simulink model "UAV_Task4_3"  (R2024b)
settings: Solver=ode45  StartTime=0  StopTime=100  RelTol=1e-5  AbsTol=1e-5
values from neighbouring files (symbols this model uses):
  adaptiveActivation = 1    [UAV_Task4_1_main.m]    (also in UAV_Task4_2_main.m = 0; UAV_Task4_3_main.m)
  B_p = 1/UAV.m    [UAV_Task4_1_main.m]    (also in UAV_Task4_2_main.m; UAV_Task4_3_main.m)
  F2plus = F2'*pinv(F2*F2')    [UAV_Task4_1_main.m]    (also in UAV_Task4_2_main.m; UAV_Task4_3_main.m)
  fe_0 = [0;0]    [UAV_Task4_3_main.m]
  Gamma_a = 1*[1 1 1 1]'    [UAV_Task4_1_main.m]    (also in UAV_Task4_2_main.m; UAV_Task4_3_main.m = 1*[1 1 1 1 1 1]')
  Gamma_a_scalar = 1    [UAV_Task4_2_main.m]    (also in UAV_Task4_3_main.m)
  gravityInAdaptiveController = 1    [UAV_Task4_1_main.m]    (also in UAV_Task4_2_main.m; UAV_Task4_3_main.m)
  k_f = 0.3379e-6    (= 3.379e-07)    [UAV_Task4_1_main.m]    (also in UAV_Task4_2_main.m; UAV_Task4_3_main.m)
  L = 10    [UAV_Task4_1_main.m]    (also in UAV_Task4_2_main.m; UAV_Task4_3_main.m)
  lambda_0 = 1    [UAV_Task4_1_main.m]    (also in UAV_Task4_2_main.m; UAV_Task4_3_main.m)
  Omega_0 = [1500 1500 1500 1500]'    [UAV_Task4_1_main.m]    (also in UAV_Task4_2_main.m; UAV_Task4_3_main.m)
  omegab_0 = [0; 0; 0]    [UAV_Task4_1_main.m]    (also in UAV_Task4_2_main.m; UAV_Task4_3_main.m)
  p_0 = [0; 0; 0]    [UAV_Task4_1_main.m]    (also in UAV_Task4_2_main.m; UAV_Task4_3_main.m)
  PO = 1    [UAV_Task4_1_main.m]    (also in UAV_Task4_2_main.m; UAV_Task4_3_main.m)
  q_0 = eul2quat([0, 0, 0]*degToRad,'ZYX')'    [UAV_Task4_1_main.m]    (also in UAV_Task4_2_main.m; UAV_Task4_3_main.m)
  scenario = 2    [UAV_Task4_1_main.m]    (also in UAV_Task4_2_main.m; UAV_Task4_3_main.m)
  theta_0 = [0.07;0.07;0.1]    [UAV_Task4_1_main.m]    (also in UAV_Task4_2_main.m; UAV_Task4_3_main.m)
  vb_0 = [0; 0; 0]    [UAV_Task4_1_main.m]    (also in UAV_Task4_2_main.m; UAV_Task4_3_main.m)
undefined symbols (not defined in the file or in its folder): adaptive_controller, ctrl, D_fv_i, dyn, e_3, epsilon_PO, fw_params_fc, g, lambda_i, par, pos, pos_pp, projection_operator, targetParams, theta_M, UAV, v_M, vel, vel_pp
libraries: slpidlib x22, matrix_library x6, aerolibutil x2, uavutilslib x1
(part 4 of 4)

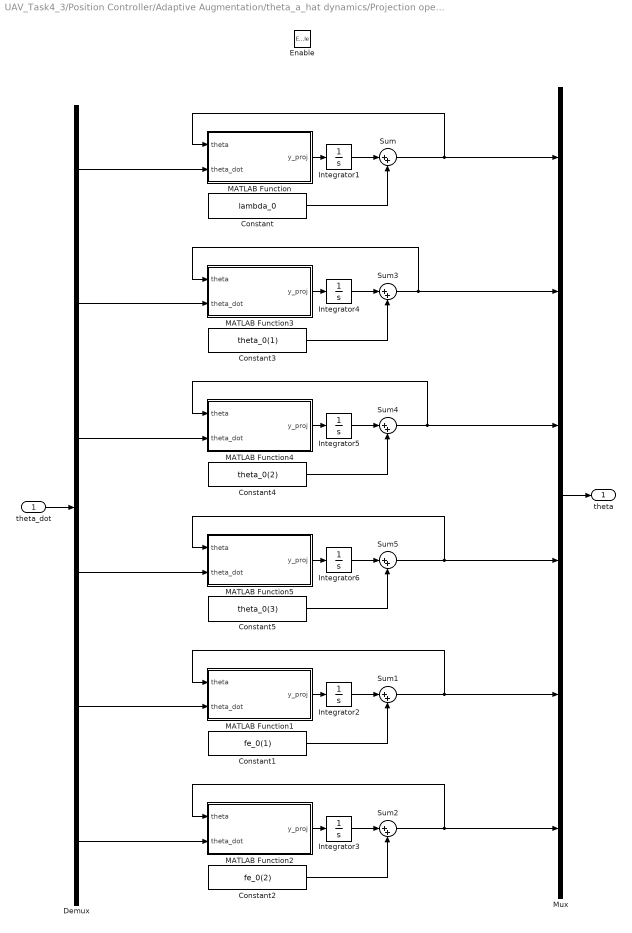
== system UAV_Task4_3/Position Controller/Adaptive Augmentation/theta_a_hat dynamics/Projection operator ==
  theta_dot : Inport
  Enable : EnablePort
  Constant : Constant  Value=lambda_0
  Constant1 : Constant  Value=fe_0(1)
  Constant2 : Constant  Value=fe_0(2)
  Constant3 : Constant  Value=theta_0(1)
  Constant4 : Constant  Value=theta_0(2)
  Constant5 : Constant  Value=theta_0(3)
  Demux : Demux  Outputs=6
  Integrator{1..6} (6 alike) : Integrator
  MATLAB Function : MATLAB Function  TreatAsAtomicUnit=on
  MATLAB Function1 : MATLAB Function  TreatAsAtomicUnit=on
  MATLAB Function2 : MATLAB Function  TreatAsAtomicUnit=on
  MATLAB Function3 : MATLAB Function  TreatAsAtomicUnit=on
  MATLAB Function4 : MATLAB Function  TreatAsAtomicUnit=on
  MATLAB Function5 : MATLAB Function  TreatAsAtomicUnit=on
  Mux : Mux  Inputs=6
  Sum{,1..5} (6 alike) : Sum  Inputs=|++
  theta : Outport
  wires:
  MATLAB Function/1(y_proj) -> Integrator1/1
  Sum/1 -> MATLAB Function/1(theta), Mux/1
  Integrator1/1 -> Sum/1
  Constant/1 -> Sum/2
  Demux/1 -> MATLAB Function/2(theta_dot)
  theta_dot/1 -> Demux/1
  Constant3/1 -> Sum3/2
  MATLAB Function3/1(y_proj) -> Integrator4/1
  Sum3/1 -> MATLAB Function3/1(theta), Mux/2
  Integrator4/1 -> Sum3/1
  Demux/2 -> MATLAB Function3/2(theta_dot)
  Constant4/1 -> Sum4/2
  MATLAB Function4/1(y_proj) -> Integrator5/1
  Sum4/1 -> MATLAB Function4/1(theta), Mux/3
  Integrator5/1 -> Sum4/1
  Demux/3 -> MATLAB Function4/2(theta_dot)
  Constant5/1 -> Sum5/2
  MATLAB Function5/1(y_proj) -> Integrator6/1
  Sum5/1 -> MATLAB Function5/1(theta), Mux/4
  Integrator6/1 -> Sum5/1
  Demux/4 -> MATLAB Function5/2(theta_dot)
  Mux/1 -> theta/1
  MATLAB Function1/1(y_proj) -> Integrator2/1
  Sum1/1 -> MATLAB Function1/1(theta), Mux/5
  Integrator2/1 -> Sum1/1
  Demux/5 -> MATLAB Function1/2(theta_dot)
  Constant1/1 -> Sum1/2
  MATLAB Function2/1(y_proj) -> Integrator3/1
  Sum2/1 -> Mux/6, MATLAB Function2/1(theta)
  Integrator3/1 -> Sum2/1
  Demux/6 -> MATLAB Function2/2(theta_dot)
  Constant2/1 -> Sum2/2

== system UAV_Task4_3/POSITION + ADAPTIVE CONTROLLER/Subsystem1/Subsystem1/Adaptive Augmentation/Predictor (x_p_hat) dynamics ==
  Lambda_hat : Inport
  u : Inport  Port=2
  phi_p : Inport  Port=3
  theta_p_hat : Inport  Port=4
  x_p : Inport  Port=5
  Add : Sum
  Constant : Constant  Value=g*e3
  Gain : Gain  Gain=B_p  Multiplication=Matrix(K*u)
  Gain1 : Gain  Gain=L
  Gain2 : Gain  Gain=gravityInAdaptiveController
  Gain3 : Gain
  Integrator : Integrator  InitialCondition=vb_0
  Matrix Multiply : Product
  Matrix Multiply1 : Product  Multiplication=Matrix(*)
  Reshape : Reshape  OutputDimensionality=Column vector (2-D)
  Reshape1 : Reshape  OutputDimensionality=Column vector (2-D)
  Reshape2 : Reshape  OutputDimensionality=Column vector (2-D)
  Scope : Scope
  Scope1 : Scope
  Sum : Sum  Inputs=+++
  Sum1 : Sum  Inputs=-+|
  Transpose : Math  Operator=transpose
  x_p_hat : Outport
  wires:
  Lambda_hat/1 -> Matrix Multiply/1
  Matrix Multiply/1 -> Add/1
  phi_p/1 -> Transpose/1
  theta_p_hat/1 -> Matrix Multiply1/2
  Matrix Multiply1/1 -> Add/2
  Add/1 -> Gain/1
  Gain/1 -> Reshape1/1
  Gain1/1 -> Reshape/1
  x_p/1 -> Scope1/1, Sum1/2
  Sum1/1 -> Gain1/1
  Integrator/1 -> Scope/1, Sum1/1, x_p_hat/1
  Sum/1 -> Integrator/1
  Reshape/1 -> Sum/1
  Reshape1/1 -> Sum/2
  Reshape2/1 -> Sum/3
  Constant/1 -> Gain2/1
  Transpose/1 -> Matrix Multiply1/1
  u/1 -> Matrix Multiply/2
  Gain2/1 -> Gain3/1
  Gain3/1 -> Reshape2/1

== system UAV_Task4_3/POSITION + ADAPTIVE CONTROLLER/Subsystem1/Subsystem1/Adaptive Augmentation/Subsystem ==
  Lambda_hat : Inport
  u_b : Inport  Port=2
  phi_p : Inport  Port=3
  theta_p_hat : Inport  Port=4
  Constant : Constant  Value=eye(3,3)
  Gain : Gain  Commented=through  Gain=-1
  Gain1 : Gain
  Inverse : MATLAB Function  TreatAsAtomicUnit=on
  Product : Product  Multiplication=Matrix(*)
  Product1 : Product  Inputs=3  Multiplication=Matrix(*)
  Subtract : Sum  Inputs=-+
  Subtract1 : Sum  Inputs=+-
  Transpose : Math  Operator=transpose
  u_a : Outport
  wires:
  Lambda_hat/1 -> Inverse/1(u)
  Inverse/1(y) -> Product1/1, Subtract/2
  Constant/1 -> Subtract/1
  Subtract/1 -> Product/1
  u_b/1 -> Product/2
  Product/1 -> Gain1/1
  Subtract1/1 -> u_a/1
  phi_p/1 -> Transpose/1
  Transpose/1 -> Gain/1
  theta_p_hat/1 -> Product1/3
  Product1/1 -> Subtract1/2
  Gain/1 -> Product1/2
  Gain1/1 -> Subtract1/1

== system UAV_Task4_3/POSITION + ADAPTIVE CONTROLLER/Subsystem1/Subsystem1/Adaptive Augmentation/phi_a ==
  u : Inport
  phi_p : Inport  Port=2
  Matrix Concatenate : Concatenate  Mode=Multidimensional array
  Scope : Scope
  Transpose : Math  Operator=transpose
  phi_a : Outport
  wires:
  Matrix Concatenate/1 -> Scope/1, phi_a/1
  u/1 -> Transpose/1
  phi_p/1 -> Matrix Concatenate/2
  Transpose/1 -> Matrix Concatenate/1

== system UAV_Task4_3/POSITION + ADAPTIVE CONTROLLER/Subsystem1/Subsystem1/Adaptive Augmentation/phi_p ==
  x_p : Inport
  Create Diagonal Matrix : matrix_library/Create Diagonal Matrix
  Gain : Gain  Gain=-1
  phi_p : Outport
  wires:
  x_p/1 -> Gain/1
  Gain/1 -> Create Diagonal Matrix/1
  Create Diagonal Matrix/1 -> phi_p/1

== system UAV_Task4_3/POSITION + ADAPTIVE CONTROLLER/Subsystem1/Subsystem1/Adaptive Augmentation/theta_a_hat dynamics ==
  Gamma_a : Inport
  phi_a : Inport  Port=2
  B_p : Inport  Port=3
  x_p : Inport  Port=4
  x_p_hat : Inport  Port=5
  Constant1 : Constant  Value=PO
  Dot Product : DotProduct  OutDataTypeStr=Inherit: Inherit via internal rule
  Integrator : Integrator  InitialCondition=[lambda_0; theta_0]
  Matrix Multiply1 : Product
  Matrix Multiply2 : Product  Multiplication=Matrix(*)
  Matrix Multiply3 : Product
  Projection operator : Subsystem
  Scope{,1..4} (5 alike) : Scope
  Sqrt : Sqrt
  Subtract : Sum  Inputs=+-
  Switch : Switch  Criteria=u2 > Threshold  SaturateOnIntegerOverflow=off  InputSameDT=off
  To Workspace : ToWorkspace  VariableName=e_p_hat  SaveFormat=Timeseries  SampleTime=-1
  Transpose : Math  Operator=transpose
  Transpose1 : Math  Commented=through  Operator=transpose
  theta_a_hat : Outport
  wires:
  x_p_hat/1 -> Subtract/2
  B_p/1 -> Transpose/1
  Subtract/1 -> Scope4/1, Dot Product/2, Dot Product/1, Matrix Multiply1/2
  Transpose/1 -> Matrix Multiply1/1
  phi_a/1 -> Transpose1/1
  Matrix Multiply1/1 -> Scope3/1, Matrix Multiply2/2
  Gamma_a/1 -> Matrix Multiply3/1
  Matrix Multiply2/1 -> Matrix Multiply3/2
  Matrix Multiply3/1 -> Projection operator/1(theta_dot), Scope2/1, Integrator/1
  x_p/1 -> Subtract/1
  Constant1/1 -> Switch/2, Projection operator/Enable
  Integrator/1 -> Scope1/1, Switch/3
  Switch/1 -> theta_a_hat/1
  Projection operator/1(theta) -> Scope/1, Switch/1
  Dot Product/1 -> Sqrt/1
  Sqrt/1 -> To Workspace/1
  Transpose1/1 -> Matrix Multiply2/1

== system UAV_Task4_3/POSITION + ADAPTIVE CONTROLLER/Subsystem1/Subsystem1/Adaptive Augmentation/theta_a_hat dynamics/Projection operator ==
  theta_dot : Inport
  Enable : EnablePort
  Constant : Constant  Value=lambda_0
  Constant3 : Constant  Value=theta_0(1)
  Constant4 : Constant  Value=theta_0(2)
  Constant5 : Constant  Value=theta_0(3)
  Demux : Demux
  Integrator{1,4..6} (4 alike) : Integrator
  MATLAB Function : MATLAB Function  TreatAsAtomicUnit=on
  MATLAB Function3 : MATLAB Function  TreatAsAtomicUnit=on
  MATLAB Function4 : MATLAB Function  TreatAsAtomicUnit=on
  MATLAB Function5 : MATLAB Function  TreatAsAtomicUnit=on
  Mux : Mux
  Sum{,3..5} (4 alike) : Sum  Inputs=|++
  theta : Outport
  wires:
  MATLAB Function/1(y_proj) -> Integrator1/1
  Sum/1 -> MATLAB Function/1(theta), Mux/1
  Integrator1/1 -> Sum/1
  Constant/1 -> Sum/2
  Demux/1 -> MATLAB Function/2(theta_dot)
  theta_dot/1 -> Demux/1
  Constant3/1 -> Sum3/2
  MATLAB Function3/1(y_proj) -> Integrator4/1
  Sum3/1 -> Mux/2, MATLAB Function3/1(theta)
  Integrator4/1 -> Sum3/1
  Demux/2 -> MATLAB Function3/2(theta_dot)
  Constant4/1 -> Sum4/2
  MATLAB Function4/1(y_proj) -> Integrator5/1
  Sum4/1 -> Mux/3, MATLAB Function4/1(theta)
  Integrator5/1 -> Sum4/1
  Demux/3 -> MATLAB Function4/2(theta_dot)
  Constant5/1 -> Sum5/2
  MATLAB Function5/1(y_proj) -> Integrator6/1
  Sum5/1 -> MATLAB Function5/1(theta), Mux/4
  Integrator6/1 -> Sum5/1
  Demux/4 -> MATLAB Function5/2(theta_dot)
  Mux/1 -> theta/1

== matlab function UAV_Task4_3/POSITION + ADAPTIVE CONTROLLER/Subsystem1/Subsystem1/Adaptive Augmentation/Subsystem/Inverse ==
  data: u input; y output
function y = fcn(u)

Lambda = diag([u;u;u]);
y = inv(Lambda);

== matlab function UAV_Task4_3/Main Trajectory Generation ==
  data: v_b_dot output size=[3,1]; v_b output size=[3,1]; p output size=[3,1]; time input; omega_p_dot output size=[3,1]; omega_p output size=[3,1]; targetParams parameter; heading output; scenario parameter
function [v_b_dot, v_b, p, omega_p_dot, omega_p, heading]   = fcn(time, targetParams, scenario)

if scenario == 1
    omega_p_dot = targetParams.omega_p_dot;
    v_b_dot = targetParams.v_b_dot;
    omega_p = targetParams.omega_p;
    v_b = targetParams.v_b;
    p = targetParams.p;
    heading = targetParams.heading;
else
    radius = norm([sqrt(2)/2 5*sqrt(2)/2 -1]);
    angle = 2*pi/60*time;
    p = [radius*sin(angle); radius*cos(angle); -1];
    v_b = pi/30*radius*[cos(angle); -sin(angle); 0];
    v_b_dot = ((pi/30*radius)^2)/3*[-sin(angle); -cos(angle); 0];
    omega_p = [0; 0; 2*pi/60];
    omega_p_dot = [0; 0; 0];
    %heading = -angle;
    heading = 0;

    % f = pi/30;
    % p = [cos(f*time) sin(f*time) -1]';
    % v_b = [-f*sin(f*time) f*cos(f*time) 0]';
    % v_b_dot = [-f^2*cos(f*time) -f^2*sin(f*time) 0]';
end

== matlab function UAV_Task4_3/Plant Dynamics/Attitude kinematics&dynamics/MATLAB Function ==
  data: quat input; quat_M output
function quat_M = fcn(quat)
qs = quat(4);

quat_M = [qs;
          quat(1) ;
          quat(2) ;
          quat(3)];

== matlab function UAV_Task4_3/POSITION + ADAPTIVE CONTROLLER/Subsystem1/Subsystem1/Adaptive Augmentation/theta_a_hat dynamics/Projection operator/MATLAB Function ==
  data: theta input; y_proj output; theta_dot input; par parameter
function y_proj = proj(theta,theta_dot,par)

% I could get rid of the center by not feeding it to the function

Gamma = par.Gamma(1);
eps_proj = par.eps_proj;
theta_M = par.theta_M(1);
center = par.center(1);
theta = theta - center;

f = 1/(eps_proj*theta_M^2)*((1+eps_proj)*(theta')*theta-theta_M^2);
grad_f = 2/(eps_proj*theta_M^2)*(1+eps_proj)*theta;

if f>0 && all(theta_dot'*Gamma*grad_f>0)
    y_proj = Gamma*theta_dot - f*Gamma*(grad_f)*grad_f'/(grad_f'*Gamma*grad_f)*Gamma*theta_dot;
else
    y_proj = Gamma*theta_dot;
end

== matlab function UAV_Task4_3/Plant Dynamics/Attitude kinematics&dynamics/Quaternion to Euler Angles1 ==
  data: quat input; euler output
function euler = quatToEuler( quat )
%	Converts a quaternion vector to ZYX Euler angles (RPY)

% quaternion is scalar first

euler = quat2eul(quat','ZYX');

end

== matlab function UAV_Task4_3/Plant Dynamics/Rigid Body dynamics&kinematics /MATLAB Function3 ==
  data: q input; R output
function R = fcn(q)

R = quat2rotm(q');

end

== matlab function UAV_Task4_3/Plant Dynamics/Attitude kinematics&dynamics/Normalization1 ==
  data: q input; q_norm output
function q_norm = quat_norm( q )

norm = sqrt( q(1)^2 + q(2)^2 + q(3)^2 + q(4)^2 );

q_norm = 1/norm * q;

== matlab function UAV_Task4_3/Position Controller/Position feedforward ==
  data: e_pos input; y output; a_d input; v_d input; v input; UAV parameter; ctrl parameter
function y = fcn(e_pos,a_d,v_d,v,UAV,ctrl)

g = 9.81;
e3 = [0; 0; 1];
m = UAV.m;
v_M = 10;

Kpos = ctrl.Kpos;

v_c_dot = - (eye(3)- diag(tanh( Kpos * e_pos/v_M).^2))*Kpos*(v-v_d) + a_d;

y = m*(v_c_dot-g*e3);

== matlab function UAV_Task4_3/Attitude Planner ==
  data: R output size=[3,3]; f_c input size=[3,1]; heading input
function R = fcn(f_c, heading)

% credo che devo mettere il - perché il mf flippa.

h_d = [cos(heading); sin(heading); 0];

k_p = -f_c/norm(f_c);

j_p = cross(k_p,h_d)/norm(cross(k_p,h_d));

i_p = cross(j_p,k_p);

R = [i_p, j_p, k_p];

== matlab function UAV_Task4_3/POSITION + ADAPTIVE CONTROLLER/Subsystem1/Subsystem1/Adaptive Augmentation/theta_a_hat dynamics/Projection operator/MATLAB Function3 ==
  data: theta input; y_proj output; theta_dot input; par parameter
function y_proj = proj(theta,theta_dot,par)

% I could get rid of the center by not feeding it to the function

Gamma = par.Gamma(2);
eps_proj = par.eps_proj;
theta_M = par.theta_M(2);
center = par.center(2);
theta = theta - center;

f = 1/(eps_proj*theta_M^2)*((1+eps_proj)*(theta')*theta-theta_M^2);
grad_f = 2/(eps_proj*theta_M^2)*(1+eps_proj)*theta;

if f>0 && all(theta_dot'*Gamma*grad_f>0)
    y_proj = Gamma*theta_dot - f*Gamma*(grad_f)*grad_f'/(grad_f'*Gamma*grad_f)*Gamma*theta_dot;
else
    y_proj = Gamma*theta_dot;
end

== matlab function UAV_Task4_3/Position Controller/Subsystem1/Subsystem1/Projection operator ==
  data: f output; theta_a_hat input; y_proj output; y input; epsilon_PO parameter; theta_M parameter; ygrad output
function [f, y_proj, ygrad] = fcn(theta_a_hat, y, epsilon_PO, theta_M)

% 1
f_1 = ((1 + epsilon_PO(1))*theta_a_hat(1)^2 - theta_M(1)^2)/(epsilon_PO(1)*theta_M(1)^2);
grad_f_1 = 2*(1 + epsilon_PO(1))*theta_a_hat(1)/(epsilon_PO(1)*theta_M(1)^2);

if f_1>0 && y(1)*grad_f_1>0
    y_proj_1 = y(1) - f_1*(grad_f_1^2)/grad_f_1^2*y(1);
else
    y_proj_1 = y(1);
end

% 2
f_2 = ((2 + epsilon_PO(2))*theta_a_hat(2)^2 - theta_M(2)^2)/(epsilon_PO(2)*theta_M(2)^2);
grad_f_2 = 2*(2 + epsilon_PO(2))*theta_a_hat(2)/(epsilon_PO(2)*theta_M(2)^2);

if f_2>0 && y(2)*grad_f_2>0
    y_proj_2 = y(2) - f_2*(grad_f_2^2)/grad_f_2^2*y(2);
else
    y_proj_2 = y(2);
end

% 3
f_3 = ((3 + epsilon_PO(3))*theta_a_hat(3)^2 - theta_M(3)^2)/(epsilon_PO(3)*theta_M(3)^2);
grad_f_3 = 2*(3 + epsilon_PO(3))*theta_a_hat(3)/(epsilon_PO(3)*theta_M(3)^2);

if f_3>0 && y(3)*grad_f_3>0
    y_proj_3 = y(3) - f_3*(grad_f_3^2)/grad_f_3^2*y(3);
else
    y_proj_3 = y(3);
end

% 4
f_4 = ((4 + epsilon_PO(4))*theta_a_hat(4)^2 - theta_M(4)^2)/(epsilon_PO(4)*theta_M(4)^2);
grad_f_4 = 2*(4 + epsilon_PO(4))*theta_a_hat(4)/(epsilon_PO(4)*theta_M(4)^2);

if f_4>0 && y(4)*grad_f_4>0
    y_proj_4 = y(4) - f_4*(grad_f_4^2)/grad_f_4^2*y(4);
else
    y_proj_4 = y(4);
end

f = [f_1, f_2, f_3, f_4]';
y_proj = [y_proj_1, y_proj_2, y_proj_3, y_proj_4]';
grad_f = [grad_f_1, grad_f_2, grad_f_3, grad_f_4]';
ygrad = [y(1)*grad_f_1, y(2)*grad_f_2, y(3)*grad_f_3, y(4)*grad_f_4];

== matlab function UAV_Task4_3/POSITION + ADAPTIVE CONTROLLER/Subsystem1/Subsystem1/Adaptive Augmentation/theta_a_hat dynamics/Projection operator/MATLAB Function4 ==
  data: theta input; y_proj output; theta_dot input; par parameter
function y_proj = proj(theta,theta_dot,par)

% I could get rid of the center by not feeding it to the function

Gamma = par.Gamma(3);
eps_proj = par.eps_proj;
theta_M = par.theta_M(3);
center = par.center(3);
theta = theta - center;

f = 1/(eps_proj*theta_M^2)*((1+eps_proj)*(theta')*theta-theta_M^2);
grad_f = 2/(eps_proj*theta_M^2)*(1+eps_proj)*theta;

if f>0 && all(theta_dot'*Gamma*grad_f>0)
    y_proj = Gamma*theta_dot - f*Gamma*(grad_f)*grad_f'/(grad_f'*Gamma*grad_f)*Gamma*theta_dot;
else
    y_proj = Gamma*theta_dot;
end

== matlab function UAV_Task4_3/POSITION + ADAPTIVE CONTROLLER/Subsystem1/Subsystem1/Adaptive Augmentation/theta_a_hat dynamics/Projection operator/MATLAB Function5 ==
  data: theta input; y_proj output; theta_dot input; par parameter
function y_proj = proj(theta,theta_dot,par)

% I could get rid of the center by not feeding it to the function

Gamma = par.Gamma(4);
eps_proj = par.eps_proj;
theta_M = par.theta_M(4);
center = par.center(4);
theta = theta - center;

f = 1/(eps_proj*theta_M^2)*((1+eps_proj)*(theta')*theta-theta_M^2);
grad_f = 2/(eps_proj*theta_M^2)*(1+eps_proj)*theta;

if f>0 && all(theta_dot'*Gamma*grad_f>0)
    y_proj = Gamma*theta_dot - f*Gamma*(grad_f)*grad_f'/(grad_f'*Gamma*grad_f)*Gamma*theta_dot;
else
    y_proj = Gamma*theta_dot;
end

== matlab function UAV_Task4_3/POSITION + ADAPTIVE CONTROLLER/Subsystem1/Subsystem1/Projection operator ==
  data: f output; theta_a_hat input; y_proj output; y input; epsilon_PO parameter; theta_M parameter; ygrad output
function [f, y_proj, ygrad] = fcn(theta_a_hat, y, epsilon_PO, theta_M)

% 1
f_1 = ((1 + epsilon_PO(1))*theta_a_hat(1)^2 - theta_M(1)^2)/(epsilon_PO(1)*theta_M(1)^2);
grad_f_1 = 2*(1 + epsilon_PO(1))*theta_a_hat(1)/(epsilon_PO(1)*theta_M(1)^2);

if f_1>0 && y(1)*grad_f_1>0
    y_proj_1 = y(1) - f_1*(grad_f_1^2)/grad_f_1^2*y(1);
else
    y_proj_1 = y(1);
end

% 2
f_2 = ((2 + epsilon_PO(2))*theta_a_hat(2)^2 - theta_M(2)^2)/(epsilon_PO(2)*theta_M(2)^2);
grad_f_2 = 2*(2 + epsilon_PO(2))*theta_a_hat(2)/(epsilon_PO(2)*theta_M(2)^2);

if f_2>0 && y(2)*grad_f_2>0
    y_proj_2 = y(2) - f_2*(grad_f_2^2)/grad_f_2^2*y(2);
else
    y_proj_2 = y(2);
end

% 3
f_3 = ((3 + epsilon_PO(3))*theta_a_hat(3)^2 - theta_M(3)^2)/(epsilon_PO(3)*theta_M(3)^2);
grad_f_3 = 2*(3 + epsilon_PO(3))*theta_a_hat(3)/(epsilon_PO(3)*theta_M(3)^2);

if f_3>0 && y(3)*grad_f_3>0
    y_proj_3 = y(3) - f_3*(grad_f_3^2)/grad_f_3^2*y(3);
else
    y_proj_3 = y(3);
end

% 4
f_4 = ((4 + epsilon_PO(4))*theta_a_hat(4)^2 - theta_M(4)^2)/(epsilon_PO(4)*theta_M(4)^2);
grad_f_4 = 2*(4 + epsilon_PO(4))*theta_a_hat(4)/(epsilon_PO(4)*theta_M(4)^2);

if f_4>0 && y(4)*grad_f_4>0
    y_proj_4 = y(4) - f_4*(grad_f_4^2)/grad_f_4^2*y(4);
else
    y_proj_4 = y(4);
end

f = [f_1, f_2, f_3, f_4]';
y_proj = [y_proj_1, y_proj_2, y_proj_3, y_proj_4]';
grad_f = [grad_f_1, grad_f_2, grad_f_3, grad_f_4]';
ygrad = [y(1)*grad_f_1, y(2)*grad_f_2, y(3)*grad_f_3, y(4)*grad_f_4];

== matlab function UAV_Task4_3/POSITION + ADAPTIVE CONTROLLER/MATLAB Function ==
  data: f_c input; T_c output
function T_c = fcn(f_c)

T_c = norm(f_c);

%T_c = -f_c(3);

== matlab function UAV_Task4_3/Plant Dynamics/Attitude kinematics&dynamics/second term  ==
  data: a input; c output; b input
function c = cross_six(a,b)

a_v = a(1:3);
a_omega = a(4:6);

cross_six = [crossmat(a_omega), zeros(3,3);
             crossmat(a_v), crossmat(a_omega)] ;

c = cross_six*b;

end

function S=crossmat(s)
S=[0  -s(3)  s(2);
    s(3)   0 -s(1);
    -s(2)  s(1)  0];
end

== matlab function UAV_Task4_3/Plant Dynamics/Gravity wrench ==
  data: R input; w_g output; UAV parameter; par parameter
function w_g = fcn(R,UAV,par)

e_3 = par.e_3;
g = par.g;

w_g = g*[UAV.m*R'*e_3; UAV.S*R'*e_3];

== matlab function UAV_Task4_3/Plant Dynamics/Attitude kinematics&dynamics/Gravity wrench ==
  data: R input; w_g output; UAV parameter; par parameter
function w_g = fcn(R,UAV,par)

e_3 = par.e_3;
g = par.g;

w_g = g*[UAV.m*R'*e_3; UAV.S*R'*e_3];

== matlab function UAV_Task4_3/Plant Dynamics/Rigid Body dynamics&kinematics /MATLAB Function4 ==
  data: a input; c output; b input
function c = cross_six(a,b)

a_v = a(1:3);
a_omega = a(4:6);

cross_six = [crossmat(a_omega), zeros(3,3);
             crossmat(a_v), crossmat(a_omega)] ;

c = cross_six*b;

end

function S=crossmat(s)
S=[0  -s(3)  s(2);
    s(3)   0 -s(1);
    -s(2)  s(1)  0];
end

== matlab function UAV_Task4_3/Plant Dynamics/Attitude kinematics&dynamics/Quaternion kinematics1 ==
  data: omega input; quat input; q_dot output
function q_dot = quat_kin(omega, quat)

p = omega(1);
q = omega(2);
r = omega(3);

OmegaPrime = - [0 -r  q;
                r  0 -p;
               -q  p  0];

W = [OmegaPrime, omega;
      -omega',     0  ];

q_dot = 0.5*W*quat;

end

== matlab function UAV_Task4_3/Plant Dynamics/Rigid Body dynamics&kinematics /MATLAB Function ==
  data: quat input; euler output
function euler = quatToEuler( quat )
%	Converts a quaternion vector to ZYX Euler angles (RPY)

euler = quat2eul(quat','XYZ');

end

== matlab function UAV_Task4_3/Plant Dynamics/Rigid Body dynamics&kinematics /MATLAB Function1 ==
  data: omega input; quat input; q_dot output
 function q_dot = quat_kin(omega, quat)
%#codegen

eta = quat(1);
eps = quat(2:4);

W=[-eps';
   skew(eps) + eta*eye(3)];

q_dot = 0.5*W*omega;

end

function S=skew(s)
S=[0  -s(3)  s(2);
    s(3)   0 -s(1);
    -s(2)  s(1)  0];
end

== matlab function UAV_Task4_3/Plant Dynamics/Rigid Body dynamics&kinematics /MATLAB Function2 ==
  data: q input; q_norm output
function q_norm = quat_norm( q )

norm = sqrt( q(1)^2 + q(2)^2 + q(3)^2 + q(4)^2 );

q_norm = 1/norm * q;

== matlab function UAV_Task4_3/CONTROL ALLOCATION/MATLAB Function1 ==
  data: Tc input; u_c output; tau_c input; F2 parameter
function u_c = fcn(Tc, tau_c, F2)

Uv = [Tc;tau_c]; % F1*uv

F2_plus = F2'/(F2*F2');

u_c = F2_plus*Uv;


end

== matlab function UAV_Task4_3/Position Controller/Adaptive Augmentation/Subsystem/Inverse ==
  data: u input; y output
function y = fcn(u)

Lambda = diag([u;u;u]);
y = inv(Lambda);

== matlab function UAV_Task4_3/Position Controller/Adaptive Augmentation/theta_a_hat dynamics/Projection operator/MATLAB Function ==
  data: theta input; y_proj output; theta_dot input; par parameter
function y_proj = proj(theta,theta_dot,par)

% I could get rid of the center by not feeding it to the function

Gamma = par.Gamma(1);
eps_proj = par.eps_proj;
theta_M = par.theta_M(1);
center = par.center(1);
theta = theta - center;

f = 1/(eps_proj*theta_M^2)*((1+eps_proj)*(theta')*theta-theta_M^2);
grad_f = 2/(eps_proj*theta_M^2)*(1+eps_proj)*theta;

if f>0 && all(theta_dot'*Gamma*grad_f>0)
    y_proj = Gamma*theta_dot - f*Gamma*(grad_f)*grad_f'/(grad_f'*Gamma*grad_f)*Gamma*theta_dot;
else
    y_proj = Gamma*theta_dot;
end

== matlab function UAV_Task4_3/Position Controller/Adaptive Augmentation/theta_a_hat dynamics/Projection operator/MATLAB Function3 ==
  data: theta input; y_proj output; theta_dot input; par parameter
function y_proj = proj(theta,theta_dot,par)

% I could get rid of the center by not feeding it to the function

Gamma = par.Gamma(2);
eps_proj = par.eps_proj;
theta_M = par.theta_M(2);
center = par.center(2);
theta = theta - center;

f = 1/(eps_proj*theta_M^2)*((1+eps_proj)*(theta')*theta-theta_M^2);
grad_f = 2/(eps_proj*theta_M^2)*(1+eps_proj)*theta;

if f>0 && all(theta_dot'*Gamma*grad_f>0)
    y_proj = Gamma*theta_dot - f*Gamma*(grad_f)*grad_f'/(grad_f'*Gamma*grad_f)*Gamma*theta_dot;
else
    y_proj = Gamma*theta_dot;
end

== matlab function UAV_Task4_3/Position Controller/Adaptive Augmentation/theta_a_hat dynamics/Projection operator/MATLAB Function4 ==
  data: theta input; y_proj output; theta_dot input; par parameter
function y_proj = proj(theta,theta_dot,par)

% I could get rid of the center by not feeding it to the function

Gamma = par.Gamma(3);
eps_proj = par.eps_proj;
theta_M = par.theta_M(3);
center = par.center(3);
theta = theta - center;

f = 1/(eps_proj*theta_M^2)*((1+eps_proj)*(theta')*theta-theta_M^2);
grad_f = 2/(eps_proj*theta_M^2)*(1+eps_proj)*theta;

if f>0 && all(theta_dot'*Gamma*grad_f>0)
    y_proj = Gamma*theta_dot - f*Gamma*(grad_f)*grad_f'/(grad_f'*Gamma*grad_f)*Gamma*theta_dot;
else
    y_proj = Gamma*theta_dot;
end

== matlab function UAV_Task4_3/Position Controller/Adaptive Augmentation/theta_a_hat dynamics/Projection operator/MATLAB Function5 ==
  data: theta input; y_proj output; theta_dot input; par parameter
function y_proj = proj(theta,theta_dot,par)

% I could get rid of the center by not feeding it to the function

Gamma = par.Gamma(4);
eps_proj = par.eps_proj;
theta_M = par.theta_M(4);
center = par.center(4);
theta = theta - center;

f = 1/(eps_proj*theta_M^2)*((1+eps_proj)*(theta')*theta-theta_M^2);
grad_f = 2/(eps_proj*theta_M^2)*(1+eps_proj)*theta;

if f>0 && all(theta_dot'*Gamma*grad_f>0)
    y_proj = Gamma*theta_dot - f*Gamma*(grad_f)*grad_f'/(grad_f'*Gamma*grad_f)*Gamma*theta_dot;
else
    y_proj = Gamma*theta_dot;
end

== matlab function UAV_Task4_3/Plant Dynamics/Attitude kinematics&dynamics/Normalization ==
  data: q input; q_norm output
function q_norm = quat_norm( q )

norm = sqrt( q(1)^2 + q(2)^2 + q(3)^2 + q(4)^2 );

q_norm = 1/norm * q;

== matlab function UAV_Task4_3/PLANT/Gravity wrench ==
  data: R input; w_g output; UAV parameter; par parameter
function w_g = fcn(R,UAV,par)

e_3 = par.e_3;
g = par.g;

w_g = g*[UAV.m*R'*e_3; UAV.S*R'*e_3];

== matlab function UAV_Task4_3/PLANT/Rigid Body dynamics&kinematics /MATLAB Function ==
  data: quat input; euler output
function euler = quatToEuler( quat )
%	Converts a quaternion vector to ZYX Euler angles (RPY)

euler = quat2eul(quat','XYZ');

end

== matlab function UAV_Task4_3/PLANT/Rigid Body dynamics&kinematics /MATLAB Function1 ==
  data: omega input; quat input; q_dot output
 function q_dot = quat_kin(omega, quat)
%#codegen

eta = quat(1);
eps = quat(2:4);

W=[-eps';
   skew(eps) + eta*eye(3)];

q_dot = 0.5*W*omega;

end

function S=skew(s)
S=[0  -s(3)  s(2);
    s(3)   0 -s(1);
    -s(2)  s(1)  0];
end

== matlab function UAV_Task4_3/PLANT/Rigid Body dynamics&kinematics /MATLAB Function2 ==
  data: q input; q_norm output
function q_norm = quat_norm( q )

norm = sqrt( q(1)^2 + q(2)^2 + q(3)^2 + q(4)^2 );

q_norm = 1/norm * q;

== matlab function UAV_Task4_3/PLANT/Rigid Body dynamics&kinematics /MATLAB Function3 ==
  data: q input; R output
function R = fcn(q)

R = quat2rotm(q');

end

== matlab function UAV_Task4_3/PLANT/Rigid Body dynamics&kinematics /MATLAB Function4 ==
  data: a input; c output; b input
function c = cross_six(a,b)

a_v = a(1:3);
a_omega = a(4:6);

cross_six = [crossmat(a_omega), zeros(3,3);
             crossmat(a_v), crossmat(a_omega)] ;

c = cross_six*b;

end

function S=crossmat(s)
S=[0  -s(3)  s(2);
    s(3)   0 -s(1);
    -s(2)  s(1)  0];
end

== matlab function UAV_Task4_3/ATTITUDE CONTROLLER/Attitude dynamics FF/feedforward ==
  data: omega_c input; omega_b input; omega_c_dot input; tau_ff output; UAV parameter
function tau_ff = fcn(omega_c, omega_b, omega_c_dot,UAV)

J = UAV.J;

temp = J * omega_b;
tau_ff = J * omega_c_dot + cross_product(omega_c, temp);


function result = cross_product(vec1, vec2)
    
    result = [
        vec1(2) * vec2(3) - vec1(3) * vec2(2);
        vec1(3) * vec2(1) - vec1(1) * vec2(3);
        vec1(1) * vec2(2) - vec1(2) * vec2(1)
    ];
end

end

== matlab function UAV_Task4_3/Plant Dynamics/Attitude kinematics&dynamics/MATLAB Function1 ==
  data: t input; y output; par parameter
function y = fcn(t, par)

e1 = [1;0;0];
e2 = [0;1;0];
fw0 = par.fw0;
fw1 = par.fw1;

if t >= 10 && t <= 30
    fe = fw0.*e1 + fw1*sin(t).*e2;
else
    fe = [0;0;0];
end

y = [fe; 0; 0; 0];

== matlab function UAV_Task4_3/ATTITUDE CONTROLLER/Attitude kinematics/Attitude controller P ==
  data: R input; R_d input; omega_d input; omega_c output; kin parameter; quat_e output
function [omega_c, quat_e] = fcn(R,R_d,omega_d,kin)

R_e = R_d'*R; % attitude error in terms of DCM

quat_e = rotm2quat(R_e);

quat_e_v = quat_e( 2:4 )';
quat_e_s = quat_e( 1 );

% Discontinuous control law

omega_c = - 2 * kin.Kp * custom_sign( quat_e_s ) * quat_e_v + R_e'*omega_d;

e_1 = [1 0 0]';
e_2 = [0 1 0]';
e_3 = [0 0 1]';

% Another control law

omega_c = -kin.Kp(1,1)*cross(R_e'*e_1,e_1) -kin.Kp(2,2)*cross(R_e'*e_2,e_2) -kin.Kp(3,3)*cross(R_e'*e_3,e_3)+ R_e'*omega_d;

% omega_c = -kin.Kp(1,1)*cross(R_e'*e_3,e_3) - kin.Kp(2,2)/2*((R_d*e_2)'*R*e_1 - (R*e_2)'*R_d*e_1)*e_3 +  R_e'*omega_d;


end

function sign = custom_sign( scalar )
%This function returns the sign of a scalar
%   sign = custom_sign( scalar )

if scalar >= 0
    sign = 1;
else
    sign = -1;
end

end

== matlab function UAV_Task4_3/Plant Dynamics/Attitude kinematics&dynamics/Quaternion kinematics ==
  data: omega input; quat input; q_dot output
 function q_dot = quat_kin(omega, quat)
%#codegen

% quaternion is scalar first

eta = quat(1);
eps = quat(2:4);

W=[-eps';
   skew(eps) + eta*eye(3)];

q_dot = 0.5*W*omega;

end

function S=skew(s)
S=[0  -s(3)  s(2);
    s(3)   0 -s(1);
    -s(2)  s(1)  0];
end

== matlab function UAV_Task4_3/Position Controller/Adaptive Augmentation/theta_a_hat dynamics/Projection operator/MATLAB Function1 ==
  data: theta input; y_proj output; theta_dot input; par parameter
function y_proj = proj(theta,theta_dot,par)

% I could get rid of the center by not feeding it to the function

Gamma = par.Gamma(5);
eps_proj = par.eps_proj;
theta_M = par.theta_M(5);
center = par.center(5);
theta = theta - center;

f = 1/(eps_proj*theta_M^2)*((1+eps_proj)*(theta')*theta-theta_M^2);
grad_f = 2/(eps_proj*theta_M^2)*(1+eps_proj)*theta;

if f>0 && all(theta_dot'*Gamma*grad_f>0)
    y_proj = Gamma*theta_dot - f*Gamma*(grad_f)*grad_f'/(grad_f'*Gamma*grad_f)*Gamma*theta_dot;
else
    y_proj = Gamma*theta_dot;
end

== matlab function UAV_Task4_3/TRAJECTORY PLANNER/Heading ==
  data: h_d output; psi parameter
function h_d = fcn(psi)

h_d = [cos(psi) sin(psi) 0]';

== matlab function UAV_Task4_3/TRAJECTORY PLANNER/Trajectory planner ==
  data: t input; p_d output; v_d output; a_d output; trajectory parameter
function [p_d, v_d, a_d] = fcn(t, trajectory)

if trajectory == 1

    f = pi/30;
    p_d= [cos(f*t) sin(f*t) -1]';
    v_d= [-f*sin(f*t) f*cos(f*t) 0]';
    a_d= [-f^2*cos(f*t) -f^2*sin(f*t) 0]';

else

    p_d = [0 2 -1]';
    v_d = [0 0 0]';
    a_d = [0 0 0]';

end

== matlab function UAV_Task4_3/Position Controller/Adaptive Augmentation/theta_a_hat dynamics/Projection operator/MATLAB Function2 ==
  data: theta input; y_proj output; theta_dot input; par parameter
function y_proj = proj(theta,theta_dot,par)

% I could get rid of the center by not feeding it to the function

Gamma = par.Gamma(6);
eps_proj = par.eps_proj;
theta_M = par.theta_M(6);
center = par.center(6);
theta = theta - center;

f = 1/(eps_proj*theta_M^2)*((1+eps_proj)*(theta')*theta-theta_M^2);
grad_f = 2/(eps_proj*theta_M^2)*(1+eps_proj)*theta;

if f>0 && all(theta_dot'*Gamma*grad_f>0)
    y_proj = Gamma*theta_dot - f*Gamma*(grad_f)*grad_f'/(grad_f'*Gamma*grad_f)*Gamma*theta_dot;
else
    y_proj = Gamma*theta_dot;
end

== matlab function UAV_Task4_3/Plant Dynamics/Attitude kinematics&dynamics/Quaternion to DCM ==
  data: quat input; A output
function A = fcn(quat)

%A = quat2rotm(quat');

%   Converts a quaternion vector to the attitude matrix A
%
%   A = quatToAtt( quat )
%
%   The quaternion must be written as a 4-by-1 vector with the scalar
%   element as the fourth component.
%   The returned attitude matrix A represents the rotational matrix from 
%   the inertial reference frame to the body frame of the vehicle.
%
%   References:
%	[1] Markley, F. Landis. "Attitude error representations for Kalman filtering." 
%       Journal of guidance control and dynamics 26.2 (2003): 311-317.

quat = quat / norm(quat);

qv = [quat(1) ;
      quat(2) ;
      quat(3)];
qs = quat(4);

rox = [   0    -qv(3)  qv(2) ;
         qv(3)   0    -qv(1) ;
        -qv(2)  qv(1)   0   ];

norm_qv_sq = qv(1)^2 + qv(2)^2 + qv(3)^2;

A = (qs^2 - norm_qv_sq) * eye(3) + 2 * (qv * qv') - 2 * qs * rox;

end

== matlab function UAV_Task4_3/Plant Dynamics/Attitude kinematics&dynamics/Quaternion to DCM1 ==
  data: q input; R output
function R = fcn(q)

% quaternion is scalar first

R = quat2rotm(q');

end

== matlab function UAV_Task4_3/Attitude Controller/Attitude controller (Kin) ==
  data: R_d input; omega_d input; R input; omega_c output; ctrl parameter; quat_e output; par parameter
function [omega_c, quat_e] = fcn(R_d,omega_d,R,ctrl,par)

e_1 = par.e_1;
e_2 = par.e_2;
e_3 = par.e_3;

R_e = R_d'*R; % attitude error in terms of DCM

% Quternion feedback (discontinuous)

quat_e = rotm2quat(R_e);

quat_e_v = quat_e( 2:4 )';
quat_e_s = quat_e( 1 );

omega_c = - 2 * ctrl.Kq * custom_sign( quat_e_s ) * quat_e_v + R_e'*omega_d;

% DCM feedback

omega_c = - ctrl.KR(1,1)*cross(R_e'*e_1,e_1) - ctrl.KR(2,2)*cross(R_e'*e_2,e_2) - ctrl.KR(3,3)*cross(R_e'*e_3,e_3) + R_e'*omega_d;

% Thrust axis prioritization (geodesic feedback)

%omega_c = -ctrl.Kq(1,1)*cross(R_e'*e_3,e_3) - ctrl.Kq(3,3)/2*((R_d*e_2)'*R*e_1 - (R*e_2)'*R_d*e_1)*e_3 +  R_e'*omega_d;


end

function sign = custom_sign( scalar )
%This function returns the sign of a scalar
%   sign = custom_sign( scalar )

if scalar >= 0
    sign = 1;
else
    sign = -1;
end

end

== matlab function UAV_Task4_3/Attitude Controller/Attitude feedforward ==
  data: omega_b input size=[3,1]; omega_c_dot input; omega_c input; tau_ff output; UAV parameter
function tau_ff = fcn(omega_b,omega_c_dot, omega_c, UAV)

J = UAV.J;

tau_ff = J*omega_c_dot + cross(omega_c,J*omega_b);  % P2L4 pag. 22

== matlab function UAV_Task4_3/Plant Dynamics/Attitude kinematics&dynamics/Quaternion to Euler Angles ==
  data: quat input; euler output
function euler = quatToEuler( quat )
%	Converts a quaternion vector to ZYX Euler angles (RPY)

% quat is scalar last
% quat1 is scalar first
quat1 = quat;
quat1(1) = quat(4);
quat1(2:4) = quat(1:3);

euler = quat2eul(quat1','XYZ');

end

== matlab function UAV_Task4_3/POSITION + ADAPTIVE CONTROLLER/POSITION CONTROLLER/Position controller/MATLAB Function1 ==
  data: p input; v input; v_c output; p_d input; v_d input; a_d input; pos parameter; a_c output; v_M parameter
function [v_c , a_c] = fcn(p, v, p_d, v_d, a_d, pos, v_M)

e_p = p - p_d;

v_c = - v_M*tanh( pos.Kp * e_p/v_M ) + v_d;

a_c = - (eye(3)- diag(tanh( pos.Kp * e_p/v_M).^2))*pos.Kp*(v-v_d) + a_d;
